simulink model "Week8Practice2"  (R2025b)
settings: Solver=VariableStepAuto  StartTime=0.0  StopTime=2  MaxStep=0.001  RelTol=1e-3
settings Model: Creator=byyn002  LastModifiedBy=Kittitouch Tantiwong

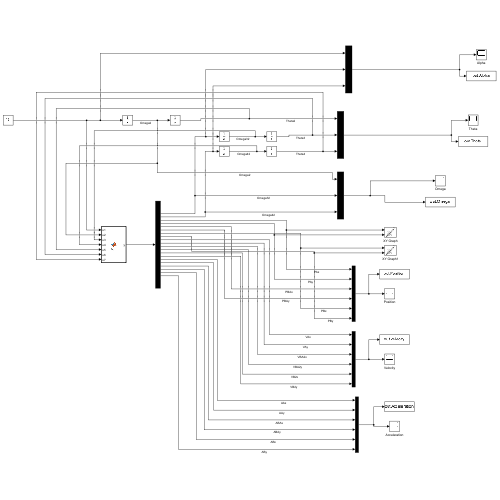
[thumbnail: Simulink's stored preview of the top-level diagram]
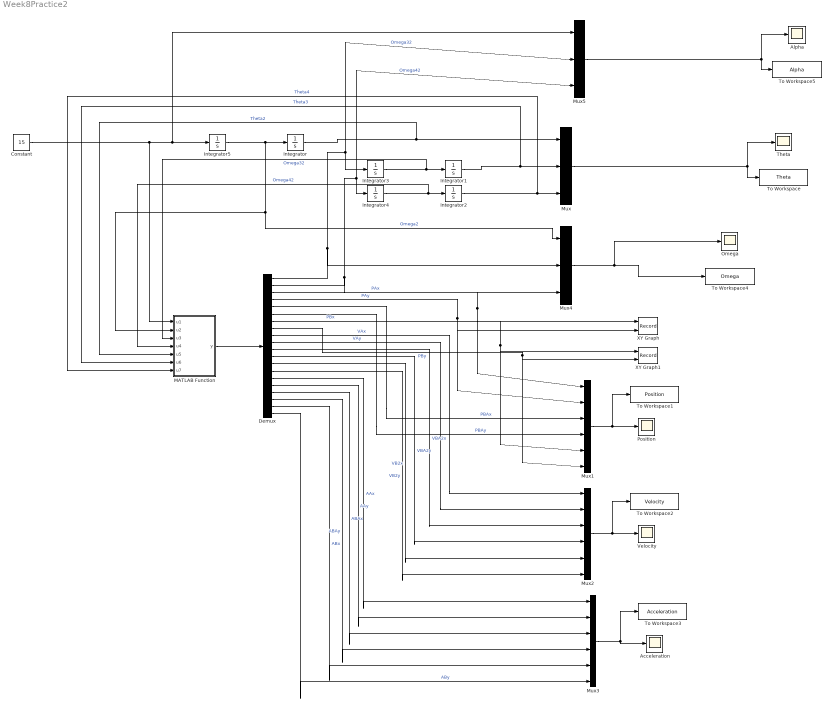
== system Week8Practice2 ==
  Acceleration : Scope
      settings: ActiveDisplayYMinimum=-441.51133  ActiveDisplayYMaximum=350.2598
  Alpha : Scope
      settings: ActiveDisplayYMinimum=-3711.79571  ActiveDisplayYMaximum=5827.18624
  Constant : Constant  Value=15
  Demux : Demux  Outputs=20
  Integrator : Integrator  InitialCondition=deg2rad(40)
  Integrator1 : Integrator  InitialCondition=deg2rad(20.2979)
  Integrator2 : Integrator  InitialCondition=deg2rad(57.3249)
  Integrator3 : Integrator  InitialCondition=-4.1209
  Integrator4 : Integrator  InitialCondition=6.9980
  Integrator5 : Integrator  InitialCondition=25
  MATLAB Function : MATLAB Function  TreatAsAtomicUnit=on
  Mux : Mux  Inputs=3
  Mux1 : Mux  Inputs=6
  Mux2 : Mux  Inputs=6
  Mux3 : Mux  Inputs=6
  Mux4 : Mux  Inputs=3
  Mux5 : Mux  Inputs=3
  Omega : Scope
      settings: ActiveDisplayYMinimum=-3711.79571  ActiveDisplayYMaximum=5827.18624  DataLoggingVariableName=ScopeData2
  Position : Scope
      settings: ActiveDisplayYMinimum=-0.06325  ActiveDisplayYMaximum=0.16925
  Theta : Scope
      settings: ActiveDisplayYMinimum=-9.73  ActiveDisplayYMaximum=90.7457
  To Workspace : ToWorkspace  VariableName=Theta  SaveFormat=Timeseries  SampleTime=-1
  To Workspace1 : ToWorkspace  VariableName=Position  SaveFormat=Timeseries  SampleTime=-1
  To Workspace2 : ToWorkspace  VariableName=Velocity  SaveFormat=Timeseries  SampleTime=-1
  To Workspace3 : ToWorkspace  VariableName=Acceleration  SaveFormat=Timeseries  SampleTime=-1
  To Workspace4 : ToWorkspace  VariableName=Omega  SaveFormat=Timeseries  SampleTime=-1
  To Workspace5 : ToWorkspace  VariableName=Alpha  SaveFormat=Timeseries  SampleTime=-1
  Velocity : Scope
      settings: ActiveDisplayYMinimum=-4.43106  ActiveDisplayYMaximum=4.99684
  XY Graph : Record  NumPorts=2.0  FileSettingsInternal="{\"entries\":[{\"content\":{\"excelSettings\":{\"content\":{},\"type\":\"Streamout.ExcelSettings\"},\"parquetSettings\":{\"content\":{},\"type\":\"Streamout.ParquetSettings\"}},\"type\":\"Streamout.FileSettingStorage\",\"uuid\":\"\"}],\"packageUris\":[\"http:\\/\\/schema.mathworks.com\\/mf0\\/streamout_blocks\\/R2020a\"],\"version\":\"1.0\"}"  FrameSettings=[0, 0]  Layout=[1 1]  SignalsInternal="{\"entries\":[{\"content\":{\"signals\":[{\"content\":{\"blockPath\":[],\"dimensions\":[1,1],\"domain\":\"\",\"lineColor\":\"#a2142f\",\"plots\":[ 1 ],\"port\":1,\"signalID\":1,\"signalName\":\"PAx\"},\"type\":\"RecordBlkView.Signal\",\"uuid\":\"\"},{\"content\":{\"blockPath\":[],\"dimensions\":[1,1],\"domain\":\"\",\"lineColor\":\"#139fff\",\"plots\":[ 1 ],\"port\":2,\"signalID\":2,\"signalName\":\"PAy\"},\"type\":\"RecordBlkView.Signal\",\"uuid\":\"\"}]},\"type\":\"RecordBlkView.InputSignals\",\"uuid\":\"\"}],\"packageUris\":[\"http:\\/\\/schema.mathworks.com\\/mf0\\/streamout_blocks\\/R2020a\"],\"version\":\"1.0\"}"  VisualizationBindings="{\"xyplotplugin\":{\"info\":[{\"series\":[{\"bindingParametersList\":[{\"parameter\":\"X-Axis\",\"signalID\":1,\"signalName\":\"PAx\"},{\"parameter\":\"Y-Axis\",\"signalID\":2,\"signalName\":\"PAy\"}],\"seriesID\":0}],\"subplotID\":1}]}}"  CompatibilityTag=XY
  XY Graph1 : Record  NumPorts=2.0  FileSettingsInternal="{\"entries\":[{\"content\":{\"excelSettings\":{\"content\":{},\"type\":\"Streamout.ExcelSettings\"},\"parquetSettings\":{\"content\":{},\"type\":\"Streamout.ParquetSettings\"}},\"type\":\"Streamout.FileSettingStorage\",\"uuid\":\"\"}],\"packageUris\":[\"http:\\/\\/schema.mathworks.com\\/mf0\\/streamout_blocks\\/R2020a\"],\"version\":\"1.0\"}"  FrameSettings=[0, 0]  Layout=[1 1]  SignalsInternal="{\"entries\":[{\"content\":{\"signals\":[{\"content\":{\"blockPath\":[],\"dimensions\":[1,1],\"domain\":\"\",\"lineColor\":\"#a2142f\",\"plots\":[ 1 ],\"port\":1,\"signalID\":1,\"signalName\":\"PBx\"},\"type\":\"RecordBlkView.Signal\",\"uuid\":\"\"},{\"content\":{\"blockPath\":[],\"dimensions\":[1,1],\"domain\":\"\",\"lineColor\":\"#139fff\",\"plots\":[ 1 ],\"port\":2,\"signalID\":2,\"signalName\":\"PBy\"},\"type\":\"RecordBlkView.Signal\",\"uuid\":\"\"}]},\"type\":\"RecordBlkView.InputSignals\",\"uuid\":\"\"}],\"packageUris\":[\"http:\\/\\/schema.mathworks.com\\/mf0\\/streamout_blocks\\/R2020a\"],\"version\":\"1.0\"}"  VisualizationBindings="{\"xyplotplugin\":{\"info\":[{\"series\":[{\"bindingParametersList\":[{\"parameter\":\"X-Axis\",\"signalID\":1,\"signalName\":\"PBx\"},{\"parameter\":\"Y-Axis\",\"signalID\":2,\"signalName\":\"PBy\"}],\"seriesID\":0}],\"subplotID\":1}]}}"  CompatibilityTag=XY
  wires:
  MATLAB Function/1(y) -> Demux/1
  Mux/1 -> To Workspace/1, Theta/1
  Demux/3 -> Mux1/1, XY Graph/1  "PAx"
  Demux/4 -> Mux1/2, XY Graph/2  "PAy"
  Demux/5 -> Mux1/3  "PBAx"
  Demux/6 -> Mux1/4  "PBAy"
  Demux/7 -> Mux1/5, XY Graph1/1  "PBx"
  Demux/8 -> Mux1/6, XY Graph1/2  "PBy"
  Mux1/1 -> To Workspace1/1, Position/1
  Integrator/1 -> MATLAB Function/5(u5), Mux/1  "Theta2"
  Integrator1/1 -> MATLAB Function/6(u6), Mux/2  "Theta3"
  Integrator2/1 -> MATLAB Function/7(u7), Mux/3  "Theta4"
  Mux2/1 -> To Workspace2/1, Velocity/1
  Demux/9 -> Mux2/1  "VAx"
  Demux/10 -> Mux2/2  "VAy"
  Demux/11 -> Mux2/3  "VBA2x"
  Demux/12 -> Mux2/4  "VBA2y"
  Demux/13 -> Mux2/5  "VB2x"
  Demux/14 -> Mux2/6  "VB2y"
  Mux3/1 -> Acceleration/1, To Workspace3/1
  Demux/15 -> Mux3/1  "AAx"
  Demux/16 -> Mux3/2  "AAy"
  Demux/17 -> Mux3/3  "ABAx"
  Demux/18 -> Mux3/4  "ABAy"
  Demux/19 -> Mux3/5  "ABx"
  Demux/20 -> Mux3/6  "ABy"
  Integrator4/1 -> MATLAB Function/4(u4), Integrator2/1  "Omega42"
  Integrator3/1 -> MATLAB Function/3(u3), Integrator1/1  "Omega32"
  Demux/2 -> Mux4/3, Mux5/3, Integrator4/1  "Omega42"
  Demux/1 -> Mux4/2, Mux5/2, Integrator3/1  "Omega32"
  Integrator5/1 -> Mux4/1, MATLAB Function/2(u2), Integrator/1  "Omega2"
  Mux4/1 -> Omega/1, To Workspace4/1
  Mux5/1 -> To Workspace5/1, Alpha/1
  Constant/1 -> Mux5/1, Integrator5/1, MATLAB Function/1(u1)

== matlab function Week8Practice2/MATLAB Function ==
  data: u1 input; y output; u2 input; u3 input; u4 input; u5 input; u6 input; u7 input
function y = fcn(u1,u2,u3,u4,u5,u6,u7)
%u1: w1
%u2:theta2 in rad
%u3: theta3 in rad
%u4: theta4 in rad

L1 = 0.1; %length of Link1 d
L2 = 0.04; %length of Link2 a
L3 = 0.12; %length of Link3 c
L4 = 0.08; %length of Link4 d
a = L2;
b = L3;
c = L4;
d = L1;

alpha2 = u1
%w2 = u1;
%q2d = rad2deg(u2);
w2 = u2;
w32 = u3;
w42 = u4;
q2 = u5; % radian angle
q32 = u6;
q42 = u7;

RA = a*exp(j*q2);
%RBA1 = b*exp(j*q31); %q31 Crossed circuit
RBA2 = b*exp(j*q32); %q32 Open circuit

%RB1 = RA + RBA1; %Position vector for Crossed circuit
RB2 = RA + RBA2; %Position vector for Open circuit

RAx = real(RA); 
RAy = imag(RA);

%RBA1x = real(RBA1); %for Crossed circuit
%RBA1y = imag(RBA1); %for Crossed circuit

RBA2x = real(RBA2);
RBA2y = imag(RBA2);

%RB1x = real(RB1); %Position Bx for Crossed circuit
%RB1y = imag(RB1); %Position By for Crossed circuit
RB2x = real(RB2); %Position Bx for Open circuit
RB2y = imag(RB2); %Position By for Open circuit

VA = j*a*w2*exp(j*q2);
VAx = real(VA);
VAy = imag(VA);
VBA2 = j*b*w32*exp(j*q32);
VBA2x = real(VBA2);
VBA2y = imag(VBA2);

%VB2 = j*c*w42*exp(j*q42);
VB =  VA + VBA2; 
VBx = real(VB);
VBy = imag(VB);
%VB2x = real(VB2);
%VB2y = imag(VB2);

%alpha2 = 15; %25 rad/sec^2

A = c*sin(q42); B = b*sin(q32);
C = a*alpha2*sin(q2)+a*w2^2*cos(q2)+b*w32^2*cos(q32)-c*w42^2*cos(q42);
D = c*cos(q42); E = b*cos(q32);
F = a*alpha2*cos(q2)-a*w2^2*sin(q2)-b*w32^2*sin(q32)+c*w42^2*sin(q42);

alpha42 = (C*E-B*F)/(A*E-B*D);
alpha32 = (C*D-A*F)/(A*E-B*D);

AA = a*alpha2*j*exp(j*q2)-a*w2^2*exp(j*q2);% polar coordinate 
AAx = real(AA); AAy = imag(AA);

ABA = b*alpha32*j*exp(j*q32)-b*w32^2*exp(j*q32);
ABAx = real(ABA); ABAy = imag(ABA);

AB = c*alpha42*j*exp(j*q42) - c*w42^2*exp(j*q42);
ABx = real(AB); ABy = imag(AB);

xout = zeros(20,1);
xout(1) = alpha32; 
xout(2) = alpha42; 
xout(3) = RAx; 
xout(4) = RAy; 
xout(5) = RBA2x; 
xout(6) = RBA2y; 
xout(7) = RB2x; 
xout(8) = RB2y; 
xout(9) = VAx; 
xout(10) = VAy; 
xout(11) = VBA2x;
xout(12) = VBA2y;
xout(13) = VBx;
xout(14) = VBy;
xout(15) = AAx;
xout(16) = AAy;
xout(17) = ABAx;
xout(18) = ABAy;
xout(19) = ABx;
xout(20) = ABy;
y = xout;
end
